simulink model "AFE_DT2_RC"  (R2013a)
settings: Solver=FixedStepDiscrete  SolverMode=SingleTasking  StartTime=0.0  StopTime=5  FixedStep=Tpas  RelTol=1e-3
InitFcn:
  | AFE_2L_RC_param_DT1
values from neighbouring files (symbols this model uses):
  Freq = 50    [AFE_2L_RC_param_DT1.m]    (also in AFE_FV_Params.m; AFE_PontHPV2.m; AFEsimplepara.m; AFEsimpleparaDT1.m)
  hys = 100    [AFE_2L_RC_param_DT1.m]    (also in AFE_FV_Params.m = 150; AFE_PontHPV2.m = 150; AFEsimplepara.m = 0.1; AFEsimpleparaDT1.m)
  I = (P+Numd(2)/Dend(1))/Ts    [AFE_2L_RC_param_DT1.m]    (also in AFE_PontHPV2.m; AFEsimpleparaDT1.m; AFEsimpleparaPV2.m; initAFE_PontHPV3.m)
  I2 = (P2+Numd2(2)/Dend2(1))/Ts2    [AFE_2L_RC_param_DT1.m]    (also in AFEsimpleparaDT1.m)
  I3 = (P3+Numd3(2)/Dend3(1))/Ts3    [AFE_2L_RC_param_DT1.m]
  Imax = 1300    [AFE_2L_RC_param_DT1.m]    (also in AFE_FV_Params.m = 1500; AFEsimpleparaDT1.m = 5000; AFEsimpleparaPV2.m = 5000)
  P = Numd(1)/Dend(1)    [AFE_2L_RC_param_DT1.m]    (also in AFE_PontHPV2.m; AFEsimpleparaDT1.m; AFEsimpleparaPV2.m; initAFE_PontHPV3.m)
  P2 = Numd2(1)/Dend2(1)    [AFE_2L_RC_param_DT1.m]    (also in AFEsimpleparaDT1.m)
  P3 = Numd3(1)/Dend3(1)    [AFE_2L_RC_param_DT1.m]
  Tpas = 5e-5    (= 5e-05)    [AFE_2L_RC_param_DT1.m]    (also in AFE_FV_Params.m; AFE_PontHPV2.m = 3e-06; AFEsimplepara.m = 1e-05; AFEsimpleparaDT1.m)
  Vac = 2000    [AFE_2L_RC_param_DT1.m]    (also in AFE_FV_Params.m; AFE_PontHPV2.m; AFEsimplepara.m; AFEsimpleparaDT1.m)
libraries: powerlib x18, powerlib_meascontrol x8, simulink x5
settings Model: Creator=LiberT  LastModifiedBy=Daniel
settings DataIOCC: SignalLoggingSaveFormat=ModelDataLogs
settings OptimizationCC: ExpressionDepthLimit=2147483647
settings DebuggingCC: MultiTaskDSMMsg=warning  MultiTaskCondExecSysMsg=none  FcnCallInpInsideContextMsg=EnableAllAsWarning  UnconnectedInputMsg=none  UnconnectedOutputMsg=none  UnconnectedLineMsg=none  StrictBusMsg=None
settings RTWCC: IncludeERTFirstTime=on

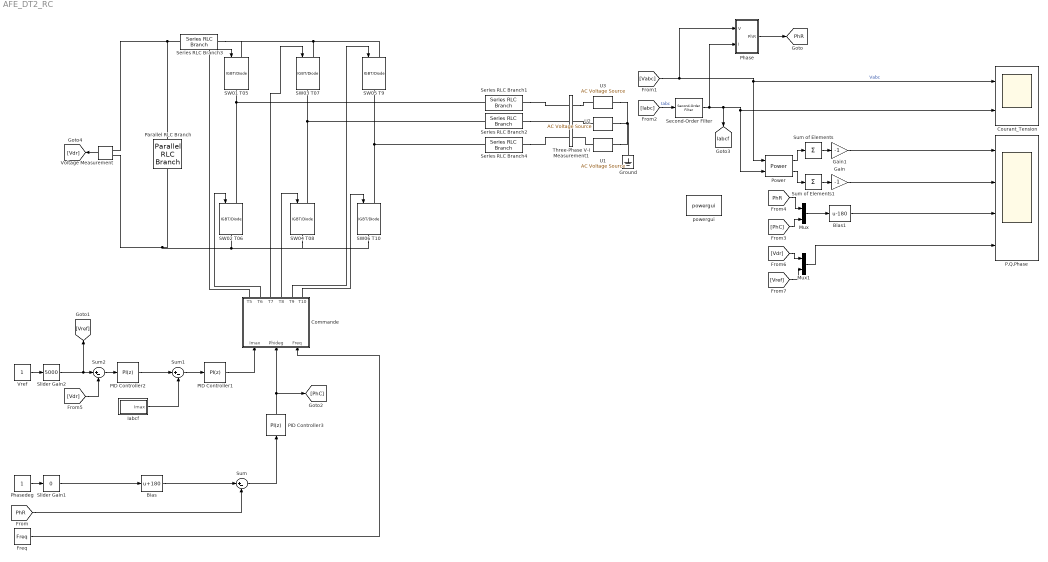
== system AFE_DT2_RC ==
  Bias : Bias  Bias=180
  Bias1 : Bias  Bias=-180
  Commande : Subsystem
  Courant_Tension : Scope  NumInputPorts=2
      settings: TickLabels=on  TimeRange=0.04  YMin=-1750~-1500  YMax=1750~1500  SaveName=Courant_Tension  MaxDataPoints=500000
  Freq : Constant  Value=Freq  SampleTime=Tpas
  Gain : Gain  Gain=-1
  Gain1 : Gain  Gain=-1
  Ground : powerlib/Elements/Ground  LConnTagsString=a
  Iabcf : Subsystem
  Mux : Mux  Inputs=2
  Mux1 : Mux  Inputs=2
  P,Q,Phase : Scope  NumInputPorts=4
      settings: TickLabels=on  TimeRange=5  YMin=0~-1.5e+06~-100~500  YMax=4e+06~4e+06~75~5500  SaveName=PQ_Phi  MaxDataPoints=500000
  PID Controller1 : simulink/Continuous/PID Controller  Controller=PI  TimeDomain=Discrete-time  SampleTime=Tpas  IntegratorMethod=Forward Euler  FilterMethod=Forward Euler  Form=Parallel  P=P2  I=I2  D=0  N=100  InitialConditionSource=internal  InitialConditionForIntegrator=0  InitialConditionForFilter=0  ExternalReset=none  LimitOutput=on  UpperSaturationLimit=1100  LowerSaturationLimit=0  LinearizeAsGain=on  AntiWindupMode=clamping  Kb=1  TrackingMode=off  Kt=1  PParamMin=[]  PParamMax=[]  IParamMin=[]  IParamMax=[]  DParamMin=[]  DParamMax=[]  NParamMin=[]  NParamMax=[]  KbParamMin=[]  KbParamMax=[]  KtParamMin=[]  KtParamMax=[]  POutMin=[]  POutMax=[]  IOutMin=[]  IOutMax=[]  DOutMin=[]  DOutMax=[]  NOutMin=[]  NOutMax=[]  KbOutMin=[]  KbOutMax=[]  KtOutMin=[]  KtOutMax=[]  IntegratorOutMin=[]  IntegratorOutMax=[]  FilterOutMin=[]  FilterOutMax=[]  SumOutMin=[]  SumOutMax=[]  SumI1OutMin=[]  SumI1OutMax=[]  SumI2OutMin=[]  SumI2OutMax=[]  SumI3OutMin=[]  SumI3OutMax=[]  SumDOutMin=[]  SumDOutMax=[]  SaturationOutMin=[]  SaturationOutMax=[]  IntegratorContinuousStateAttributes=''  IntegratorStateMustResolveToSignalObject=off  IntegratorRTWStateStorageClass=Auto  FilterContinuousStateAttributes=''  FilterStateMustResolveToSignalObject=off  FilterRTWStateStorageClass=Auto
  PID Controller2 : simulink/Continuous/PID Controller  Controller=PI  TimeDomain=Discrete-time  SampleTime=Tpas  IntegratorMethod=Forward Euler  FilterMethod=Forward Euler  Form=Parallel  P=P3  I=I3  D=0  N=100  InitialConditionSource=internal  InitialConditionForIntegrator=0  InitialConditionForFilter=0  ExternalReset=none  LimitOutput=on  UpperSaturationLimit=Imax  LowerSaturationLimit=0  LinearizeAsGain=on  AntiWindupMode=clamping  Kb=1  TrackingMode=off  Kt=1  PParamMin=[]  PParamMax=[]  IParamMin=[]  IParamMax=[]  DParamMin=[]  DParamMax=[]  NParamMin=[]  NParamMax=[]  KbParamMin=[]  KbParamMax=[]  KtParamMin=[]  KtParamMax=[]  POutMin=[]  POutMax=[]  IOutMin=[]  IOutMax=[]  DOutMin=[]  DOutMax=[]  NOutMin=[]  NOutMax=[]  KbOutMin=[]  KbOutMax=[]  KtOutMin=[]  KtOutMax=[]  IntegratorOutMin=[]  IntegratorOutMax=[]  FilterOutMin=[]  FilterOutMax=[]  SumOutMin=[]  SumOutMax=[]  SumI1OutMin=[]  SumI1OutMax=[]  SumI2OutMin=[]  SumI2OutMax=[]  SumI3OutMin=[]  SumI3OutMax=[]  SumDOutMin=[]  SumDOutMax=[]  SaturationOutMin=[]  SaturationOutMax=[]  IntegratorContinuousStateAttributes=''  IntegratorStateMustResolveToSignalObject=off  IntegratorRTWStateStorageClass=Auto  FilterContinuousStateAttributes=''  FilterStateMustResolveToSignalObject=off  FilterRTWStateStorageClass=Auto
  PID Controller3 : simulink/Continuous/PID Controller  Controller=PI  TimeDomain=Discrete-time  SampleTime=Tpas  IntegratorMethod=Forward Euler  FilterMethod=Forward Euler  Form=Parallel  P=P  I=I  D=0  N=100  InitialConditionSource=internal  InitialConditionForIntegrator=0  InitialConditionForFilter=0  ExternalReset=none  LimitOutput=on  UpperSaturationLimit=235  LowerSaturationLimit=115  LinearizeAsGain=on  AntiWindupMode=clamping  Kb=1  TrackingMode=off  Kt=1  PParamMin=[]  PParamMax=[]  IParamMin=[]  IParamMax=[]  DParamMin=[]  DParamMax=[]  NParamMin=[]  NParamMax=[]  KbParamMin=[]  KbParamMax=[]  KtParamMin=[]  KtParamMax=[]  POutMin=[]  POutMax=[]  IOutMin=[]  IOutMax=[]  DOutMin=[]  DOutMax=[]  NOutMin=[]  NOutMax=[]  KbOutMin=[]  KbOutMax=[]  KtOutMin=[]  KtOutMax=[]  IntegratorOutMin=[]  IntegratorOutMax=[]  FilterOutMin=[]  FilterOutMax=[]  SumOutMin=[]  SumOutMax=[]  SumI1OutMin=[]  SumI1OutMax=[]  SumI2OutMin=[]  SumI2OutMax=[]  SumI3OutMin=[]  SumI3OutMax=[]  SumDOutMin=[]  SumDOutMax=[]  SaturationOutMin=[]  SaturationOutMax=[]  IntegratorContinuousStateAttributes=''  IntegratorStateMustResolveToSignalObject=off  IntegratorRTWStateStorageClass=Auto  FilterContinuousStateAttributes=''  FilterStateMustResolveToSignalObject=off  FilterRTWStateStorageClass=Auto
  Parallel RLC Branch : powerlib/Elements/Parallel RLC Branch  LConnTagsString=a  RConnTagsString=__new0  BranchType=RC  Resistance=9.26  Inductance=1e-3  SetiL0=off  InitialCurrent=0  Capacitance=330e-3  Setx0=off  InitialVoltage=5000  Measurements=Branch voltage
  Phase : Subsystem
  Phasedeg : Constant  SampleTime=Tpas
  Power : powerlib_meascontrol/Measurements/Power  Freq=50  Vinit=[0, 0]  Iinit=[0, 0]  Ts=Tpas
  SW01 T05 : powerlib/Power Electronics/IGBT//Diode  Ron=1e-3  Rs=1e5  Cs=Tpas  Measurements=off
  SW02 T06 : powerlib/Power Electronics/IGBT//Diode  Ron=1e-3  Rs=1e5  Cs=Tpas  Measurements=off
  SW03 T07 : powerlib/Power Electronics/IGBT//Diode  Ron=1e-3  Rs=1e5  Cs=Tpas  Measurements=off
  SW04 T08 : powerlib/Power Electronics/IGBT//Diode  Ron=1e-3  Rs=1e5  Cs=Tpas  Measurements=off
  SW05 T9 : powerlib/Power Electronics/IGBT//Diode  Ron=1e-3  Rs=1e5  Cs=Tpas  Measurements=off
  SW06 T10 : powerlib/Power Electronics/IGBT//Diode  Ron=1e-3  Rs=1e5  Cs=Tpas  Measurements=off
  Second-Order Filter : powerlib_meascontrol/Filters/Second-Order Filter  FilterType=Bandpass  Fo=50  Zeta=0.02  Ts=Tpas  Initialize=off  Vac_Init="[0,  0,  60]"  Vdc_Init=0  PlotResponse=off  FreqRange=[0, 500, 1]
  Series RLC Branch1 : powerlib/Elements/Series RLC Branch  LConnTagsString=__new0  RConnTagsString=__new0  BranchType=L  Resistance=1  Inductance=3e-3  SetiL0=off  InitialCurrent=0  Capacitance=1e-6  Setx0=off  InitialVoltage=0  Measurements=None
  Series RLC Branch2 : powerlib/Elements/Series RLC Branch  LConnTagsString=__new0  RConnTagsString=__new0  BranchType=L  Resistance=1  Inductance=3e-3  SetiL0=off  InitialCurrent=0  Capacitance=1e-6  Setx0=off  InitialVoltage=0  Measurements=None
  Series RLC Branch3 : powerlib/Elements/Series RLC Branch  LConnTagsString=__new0  RConnTagsString=__new0  BranchType=L  Resistance=1  Inductance=5e-3  SetiL0=off  InitialCurrent=0  Capacitance=1e-6  Setx0=off  InitialVoltage=0  Measurements=None
  Series RLC Branch4 : powerlib/Elements/Series RLC Branch  LConnTagsString=__new0  RConnTagsString=__new0  BranchType=L  Resistance=1  Inductance=3e-3  SetiL0=off  InitialCurrent=0  Capacitance=1e-6  Setx0=off  InitialVoltage=0  Measurements=None
  Slider Gain1 : simulink/Math Operations/Slider Gain  low=-180  gain=0  high=180
  Slider Gain2 : simulink/Math Operations/Slider Gain  low=0  gain=5000  high=5000
  Sum : Sum  Inputs=|+-
  Sum of Elements : Sum  Inputs=+
  Sum of Elements1 : Sum  Inputs=+
  Sum1 : Sum  Inputs=|+-
  Sum2 : Sum  Inputs=|+-
  Three-Phase V-I Measurement1 : powerlib/Measurements/Three-Phase V-I Measurement  VoltageMeasurement=phase-to-ground  SetLabelV=on  LabelV=Vabc  Vpu=off  VpuLL=off  CurrentMeasurement=yes  SetLabelI=on  LabelI=Iabc  Ipu=off  Pbase=100e6  Vbase=500e3  OutputType=Complex  PhasorSimulation=off  PSBequivalent=0
  U1 : powerlib/Electrical Sources/AC Voltage Source  Amplitude=Vac*sqrt(2/3)  Phase=120  Frequency=Freq  SampleTime=Tpas  Measurements=Voltage
  U2 : powerlib/Electrical Sources/AC Voltage Source  Amplitude=Vac*sqrt(2/3)  Phase=-120  Frequency=Freq  SampleTime=Tpas  Measurements=Voltage
  U3 : powerlib/Electrical Sources/AC Voltage Source  Amplitude=Vac*sqrt(2/3)  Phase=0  Frequency=Freq  SampleTime=Tpas  Measurements=Voltage
  Voltage Measurement : powerlib/Measurements/Voltage Measurement  PhasorSimulation=off  OutputType=Complex  PSBequivalent=0
  Vref : Constant  SampleTime=Tpas
  powergui : powerlib/powergui  Priority=1  SimulationMode=Discrete  SolverType=Tustin  SampleTime=Tpas  frequency=50  SPID=off  DisableSnubberDevices=off  DisableRonSwitches=off  DisableVfSwitches=off  SwTol=0  Interpol=off  DisplayEquations=off  frequencyindice=50  Pbase=100e6  ErrMax=1e-4  Iterations=50  UnitsV=kV  UnitsW=MW  FunctionMessages=off  echomessages=off  HookPort=off  EnableUseOfTLC=off  x0status=blocks  RestoreLinks=warning  ResistiveCurrentMeasurement=off  Frange=[0:2:500]  Ylog=off  Xlog=on  ShowGrid=off  save=off  variable=ZData  structure=ScopeData1  ZoomFFT=off  StartTime=8  cycles=100  DisplayStyle=1  fundamental=50  FreqAxis=off  MaxFrequency=100  frequencyindicesteady=1  RmsSteady=1  display=off  Ts=0  methode=off
  tag scope: Iabcf=global, PhR=global
  wires:
  [Iabc] -> Second-Order Filter/1  "Iabc"
  Commande/1(T5) -> SW01 T05/1
  Commande/2(T6) -> SW02 T06/1
  Commande/4(T8) -> SW04 T08/1
  Commande/3(T7) -> SW03 T07/1
  Commande/6(T10) -> SW06 T10/1
  Commande/5(T9) -> SW05 T9/1
  [Vabc] -> Phase/1(V), Power/1, Courant_Tension/1  "Vabc"
  Second-Order Filter/1 -> Phase/2(I), [Iabcf], Courant_Tension/2, Power/2
  Voltage Measurement/1 -> [Vdr]
  Power/1 -> Sum of Elements/1
  Power/2 -> Sum of Elements1/1
  Freq/1 -> Commande/3(Freq)
  Phasedeg/1 -> Slider Gain1/1
  [PhC] -> Mux/2
  Mux/1 -> Bias1/1
  Iabcf/1(Imax) -> Sum1/2
  PID Controller1/1 -> Commande/1(Imax)
  [Vdr] -> Sum2/2
  Vref/1 -> Slider Gain2/1
  Sum2/1 -> PID Controller2/1
  PID Controller2/1 -> Sum1/1
  [Vdr] -> Mux1/1
  [Vref] -> Mux1/2
  Mux1/1 -> P,Q,Phase/4
  Sum of Elements/1 -> Gain1/1
  Sum of Elements1/1 -> Gain/1
  Gain/1 -> P,Q,Phase/2
  Gain1/1 -> P,Q,Phase/1
  Slider Gain2/1 -> [Vref], Sum2/1
  Sum1/1 -> PID Controller1/1
  [PhR] -> Sum/2
  Slider Gain1/1 -> Bias/1
  [PhR] -> Mux/1
  Sum/1 -> PID Controller3/1
  PID Controller3/1 -> [PhC], Commande/2(Phideg)
  Phase/1(PhR) -> [PhR]
  Bias/1 -> Sum/1
  Bias1/1 -> P,Q,Phase/3
  connections:
  SW06 T10/RConn1 -- SW04 T08/RConn1 -- Voltage Measurement/LConn2 -- Parallel RLC Branch/RConn1 -- SW02 T06/RConn1
  U2/LConn1 -- U1/LConn1 -- Ground/LConn1 -- U3/LConn1
  Three-Phase V-I Measurement1/RConn1 -- U3/RConn1
  U2/RConn1 -- Three-Phase V-I Measurement1/RConn2
  U1/RConn1 -- Three-Phase V-I Measurement1/RConn3
  SW02 T06/LConn1 -- Series RLC Branch1/LConn1 -- SW01 T05/RConn1
  SW04 T08/LConn1 -- Series RLC Branch2/LConn1 -- SW03 T07/RConn1
  SW06 T10/LConn1 -- Series RLC Branch4/LConn1 -- SW05 T9/RConn1
  Series RLC Branch3/LConn1 -- Parallel RLC Branch/LConn1 -- Voltage Measurement/LConn1
  Series RLC Branch1/RConn1 -- Three-Phase V-I Measurement1/LConn1
  Series RLC Branch2/RConn1 -- Three-Phase V-I Measurement1/LConn2
  Series RLC Branch4/RConn1 -- Three-Phase V-I Measurement1/LConn3
  SW05 T9/LConn1 -- Series RLC Branch3/RConn1 -- SW01 T05/LConn1 -- SW03 T07/LConn1

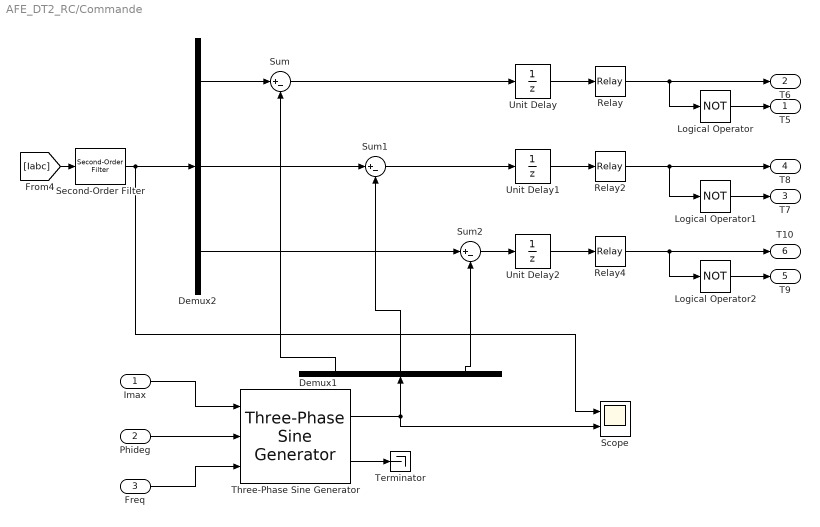
== system AFE_DT2_RC/Commande ==
  Imax : Inport
  Phideg : Inport  Port=2
  Freq : Inport  Port=3
  Demux1 : Demux  Outputs=3
  Demux2 : Demux  Outputs=3
  Logical Operator : Logic  Operator=NOT  AllPortsSameDT=off
  Logical Operator1 : Logic  Operator=NOT  AllPortsSameDT=off
  Logical Operator2 : Logic  Operator=NOT  AllPortsSameDT=off
  Relay : Relay  OnSwitchValue=hys  OffSwitchValue=-hys
  Relay2 : Relay  OnSwitchValue=hys  OffSwitchValue=-hys
  Relay4 : Relay  OnSwitchValue=hys  OffSwitchValue=-hys
  Scope : Scope  NumInputPorts=2
      settings: YMin=-1750~-1500  YMax=1750~1500
  Second-Order Filter : powerlib_meascontrol/Filters/Second-Order Filter  FilterType=Bandpass  Fo=50  Zeta=0.02  Ts=Tpas  Initialize=off  Vac_Init="[0,  0,  60]"  Vdc_Init=0  PlotResponse=off  FreqRange=[0, 500, 1]
  Sum : Sum  Inputs=|+-
  Sum1 : Sum  Inputs=|+-
  Sum2 : Sum  Inputs=|+-
  Terminator : Terminator
  Three-Phase Sine Generator : powerlib_meascontrol/Pulse & Signal Generators/Three-Phase Sine Generator  Ts=Tpas
  Unit Delay : UnitDelay  SampleTime=-1
  Unit Delay1 : UnitDelay  SampleTime=-1
  Unit Delay2 : UnitDelay  SampleTime=-1
  T5 : Outport
  T6 : Outport  Port=2
  T7 : Outport  Port=3
  T8 : Outport  Port=4
  T9 : Outport  Port=5
  T10 : Outport  Port=6
  wires:
  Demux2/1 -> Sum/1
  Demux2/2 -> Sum1/1
  Demux2/3 -> Sum2/1
  Sum/1 -> Unit Delay/1
  Sum1/1 -> Unit Delay1/1
  Sum2/1 -> Unit Delay2/1
  Unit Delay/1 -> Relay/1
  Unit Delay1/1 -> Relay2/1
  Unit Delay2/1 -> Relay4/1
  Logical Operator/1 -> T5/1
  Logical Operator1/1 -> T7/1
  Logical Operator2/1 -> T9/1
  Relay/1 -> T6/1, Logical Operator/1
  Relay2/1 -> T8/1, Logical Operator1/1
  Relay4/1 -> T10/1, Logical Operator2/1
  [Iabc] -> Second-Order Filter/1
  Imax/1 -> Three-Phase Sine Generator/1
  Demux1/2 -> Sum1/2
  Demux1/3 -> Sum2/2
  Three-Phase Sine Generator/2 -> Terminator/1
  Phideg/1 -> Three-Phase Sine Generator/2
  Demux1/1 -> Sum/2
  Three-Phase Sine Generator/1 -> Demux1/1, Scope/2
  Freq/1 -> Three-Phase Sine Generator/3
  Second-Order Filter/1 -> Scope/1, Demux2/1

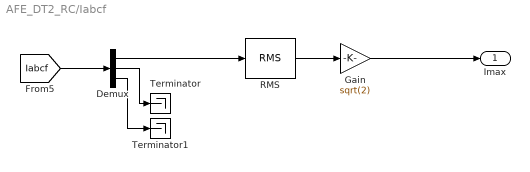
== system AFE_DT2_RC/Iabcf ==
  Demux : Demux  Outputs=3
  Gain : Gain  Gain=sqrt(2)  SampleTime=Tpas
  RMS : powerlib_meascontrol/Measurements/RMS  TrueRMS=on  Freq=Freq  RMSInit=0  Ts=Tpas
  Terminator : Terminator
  Terminator1 : Terminator
  Imax : Outport
  wires:
  [Iabcf] -> Demux/1
  Demux/3 -> Terminator1/1
  Demux/2 -> Terminator/1
  Demux/1 -> RMS/1
  RMS/1 -> Gain/1
  Gain/1 -> Imax/1

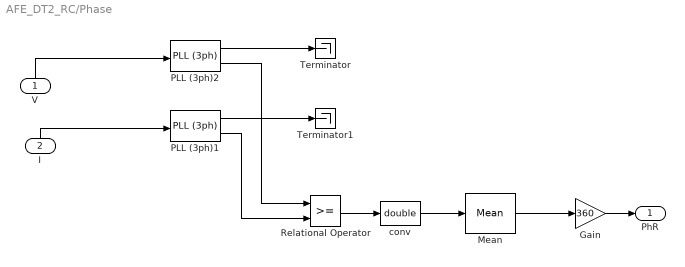
== system AFE_DT2_RC/Phase ==
  V : Inport
  I : Inport  Port=2
  Gain : Gain  Gain=360
  Mean : powerlib_meascontrol/Measurements/Mean  Freq=10  Vinit=0  Ts=Tpas
  PLL (3ph)1 : powerlib_meascontrol/PLL/PLL (3ph)  Fmin=45  Par_Init=[0, 50]  ParK=[180, 3200, 1]  TcD=1e-4  MaxRateChangeFreq=12  FilterCutOffFreq=25  Ts=Tpas  AGC=on
  PLL (3ph)2 : powerlib_meascontrol/PLL/PLL (3ph)  Fmin=45  Par_Init=[0, 50]  ParK=[180, 3200, 1]  TcD=1e-4  MaxRateChangeFreq=12  FilterCutOffFreq=25  Ts=Tpas  AGC=on
  Relational Operator : RelationalOperator  OutDataTypeStr=boolean  SampleTime=Tpas
  Terminator : Terminator
  Terminator1 : Terminator
  conv : DataTypeConversion  OutDataTypeStr=double
  PhR : Outport
  wires:
  PLL (3ph)1/2 -> Relational Operator/2
  PLL (3ph)2/1 -> Terminator/1
  PLL (3ph)2/2 -> Relational Operator/1
  I/1 -> PLL (3ph)1/1
  PLL (3ph)1/1 -> Terminator1/1
  V/1 -> PLL (3ph)2/1
  Mean/1 -> Gain/1
  Relational Operator/1 -> conv/1
  conv/1 -> Mean/1
  Gain/1 -> PhR/1
